simulink model "OfficeChairIntegratorsMarcelM"  (R2023b)
settings: Solver=VariableStepAuto  StartTime=0.0  StopTime=10.0  RelTol=1e-3
values from neighbouring files (symbols this model uses):
  b = 4000    [FindSpringConstantMarcelMartens.m]    (also in SimOfficeChairIntegratorsMarcelM.m = 2400; SimOfficeChairStateMarcelM.m = 2400)
  g = 9.82    [FindSpringConstantMarcelMartens.m]    (also in SimOfficeChairIntegratorsMarcelM.m; SimOfficeChairStateMarcelM.m)
  k = k - 10    (= 20000)    [FindSpringConstantMarcelMartens.m]    (also in SimOfficeChairIntegratorsMarcelM.m = 21610; SimOfficeChairStateMarcelM.m = 21610)
  m = 5    [FindSpringConstantMarcelMartens.m]    (also in SimOfficeChairIntegratorsMarcelM.m; SimOfficeChairStateMarcelM.m)
  M = 75    [FindSpringConstantMarcelMartens.m]    (also in SimOfficeChairIntegratorsMarcelM.m; SimOfficeChairStateMarcelM.m)
settings Model: Creator=marcelmartens  LastModifiedBy=marcelmartens

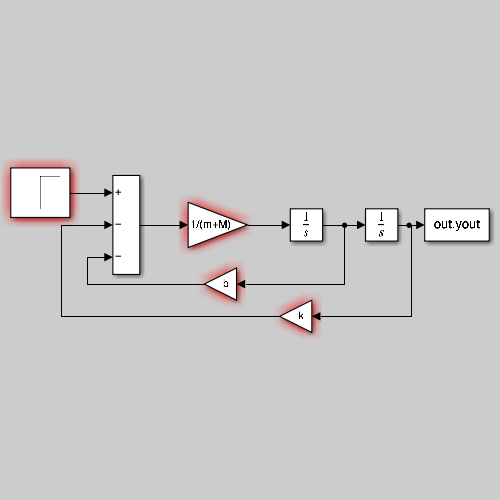
[thumbnail: Simulink's stored preview of the top-level diagram]
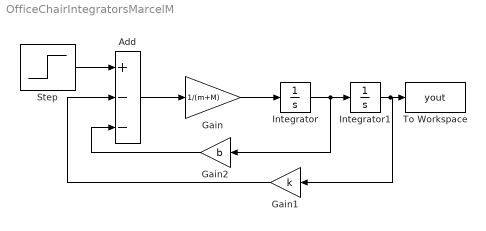
== system OfficeChairIntegratorsMarcelM ==
  Add : Sum  Inputs=+--
  Gain : Gain  Gain=1/(m+M)
  Gain1 : Gain  Gain=k
  Gain2 : Gain  Gain=b
  Integrator : Integrator
  Integrator1 : Integrator
  Step : Step  Time=0  After=M*g  SampleTime=0
  To Workspace : ToWorkspace  VariableName=yout  SaveFormat=Timeseries  SampleTime=-1
  wires:
  Integrator1/1 -> To Workspace/1, Gain1/1
  Integrator/1 -> Integrator1/1, Gain2/1
  Step/1 -> Add/1
  Gain1/1 -> Add/2
  Gain/1 -> Integrator/1
  Gain2/1 -> Add/3
  Add/1 -> Gain/1
